simulink model "porte_avion_model"  (R2025a)
settings: Solver=VariableStepAuto  StartTime=0.0  StopTime=30  RelTol=1e-3
values from neighbouring files (symbols this model uses):
  a = 250e3    (= 250000)    [bateau_data.m]    (also in chariot_data.m; porte_avion.m)
  A = [0    1  0    0 ... (first row only)    [porte_avion.m]
  b = 1e9    (= 1000000000)    [bateau_data.m]    (also in chariot_data.m; porte_avion.m)
  B = [0 ... (first row only)    [porte_avion.m]
  c = 0.4e9    (= 400000000)    [bateau_data.m]    (also in chariot_data.m; porte_avion.m)
  C = [1 0 0 0 ... (first row only)    [porte_avion.m]
  d = 500e6    (= 500000000)    [bateau_data.m]    (also in chariot_data.m; porte_avion.m)
  D = [0 ... (first row only)    [porte_avion.m]
  f = 60    [bateau_data.m]    (also in chariot_data.m; porte_avion.m)
  g = 9.81    [bateau_data.m]    (also in chariot_data.m; porte_avion.m)
  theta_0 = pi/3    (= 1.0471975512)    [porte_avion.m]
  theta_dot_0 = 0    [porte_avion.m]
  x_0 = 0    [porte_avion.m]
  X_0 = [x_0 ... (first row only)    [porte_avion.m]
  x_dot_0 = 0    [porte_avion.m]
settings Model: Creator=vikfo  LastModifiedBy=vikfo

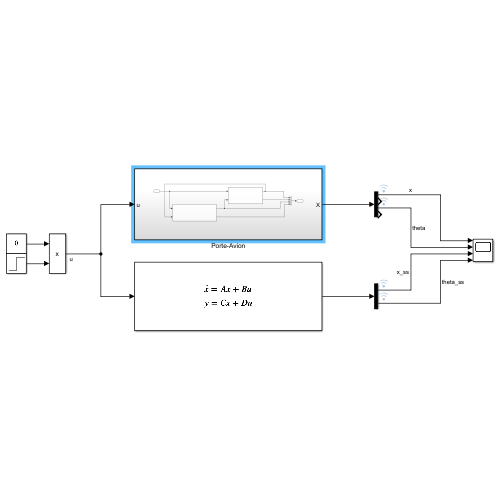
[thumbnail: Simulink's stored preview of the top-level diagram]
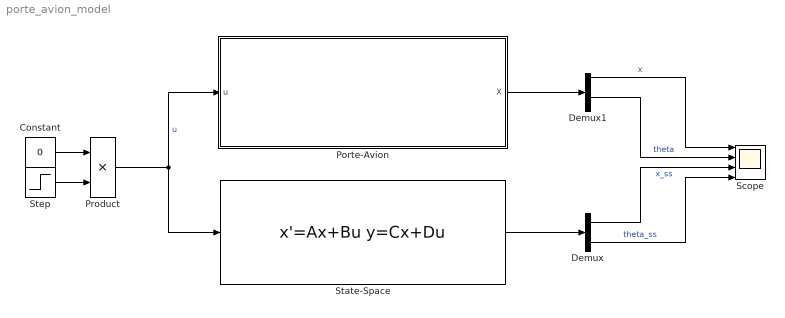
== system porte_avion_model ==
  Constant : Constant  Value=0
  Demux : Demux  Outputs=2
  Demux1 : Demux
  Porte-Avion : Subsystem
  Product : Product
  Scope : Scope  NumInputPorts=4
      settings: ActiveDisplayYMinimum=-1  ActiveDisplayYMaximum=1
  State-Space : StateSpace  A=A  B=B  C=C  D=D  InitialCondition=X_0
  Step : Step  SampleTime=0
  wires:
  Step/1 -> Product/2
  Constant/1 -> Product/1
  State-Space/1 -> Demux/1
  Demux/1 -> Scope/3  "x_ss"
  Product/1 -> Porte-Avion/1(u), State-Space/1  "u"
  Porte-Avion/1(X) -> Demux1/1
  Demux/2 -> Scope/4  "theta_ss"
  Demux1/1 -> Scope/1  "x"
  Demux1/3 -> Scope/2  "theta"

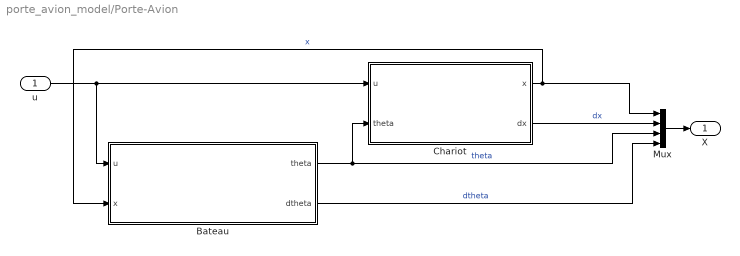
== system porte_avion_model/Porte-Avion ==
  u : Inport
  Bateau : Subsystem
  Chariot : Subsystem
  Mux : Mux
  X : Outport
  wires:
  Chariot/1(x) -> Bateau/2(x), Mux/1  "x"
  Bateau/1(theta) -> Mux/3, Chariot/2(theta)  "theta"
  Chariot/2(dx) -> Mux/2  "dx"
  u/1 -> Chariot/1(u), Bateau/1(u)
  Bateau/2(dtheta) -> Mux/4  "dtheta"
  Mux/1 -> X/1

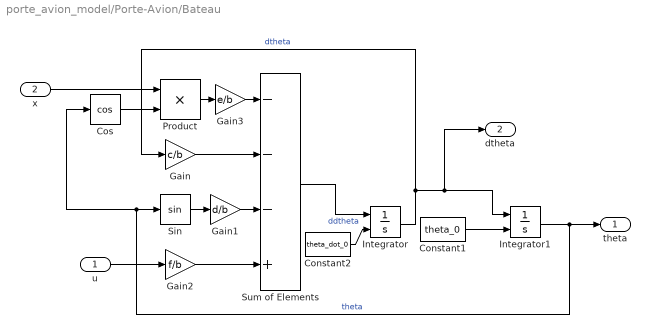
== system porte_avion_model/Porte-Avion/Bateau ==
  u : Inport
  x : Inport  Port=2
  Constant1 : Constant  Value=theta_0
  Constant2 : Constant  Value=theta_dot_0
  Cos : Trigonometry  Operator=cos
  Gain : Gain  Gain=c/b
  Gain1 : Gain  Gain=d/b
  Gain2 : Gain  Gain=f/b
  Gain3 : Gain  Gain=e/b
  Integrator : Integrator  InitialConditionSource=external
  Integrator1 : Integrator  InitialConditionSource=external
  Product : Product
  Sin : Trigonometry
  Sum of Elements : Sum  Inputs=---+
  theta : Outport
  dtheta : Outport  Port=2
  wires:
  Integrator/1 -> Gain/1, dtheta/1, Integrator1/1  "dtheta"
  u/1 -> Gain2/1
  Sum of Elements/1 -> Integrator/1  "ddtheta"
  Gain/1 -> Sum of Elements/2
  Gain2/1 -> Sum of Elements/4
  Integrator1/1 -> Cos/1, Sin/1, theta/1  "theta"
  Gain1/1 -> Sum of Elements/3
  Constant1/1 -> Integrator1/2
  Sin/1 -> Gain1/1
  Constant2/1 -> Integrator/2
  Gain3/1 -> Sum of Elements/1
  Product/1 -> Gain3/1
  x/1 -> Product/1
  Cos/1 -> Product/2

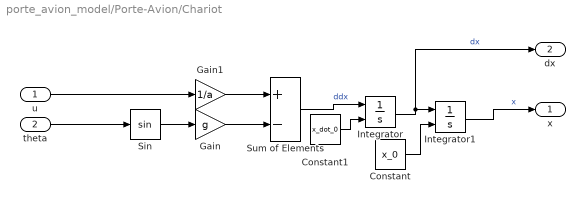
== system porte_avion_model/Porte-Avion/Chariot ==
  u : Inport
  theta : Inport  Port=2
  Constant : Constant  Value=x_0
  Constant1 : Constant  Value=x_dot_0
  Gain : Gain  Gain=g
  Gain1 : Gain  Gain=1/a
  Integrator : Integrator  InitialConditionSource=external
  Integrator1 : Integrator  InitialConditionSource=external
  Sin : Trigonometry
  Sum of Elements : Sum  Inputs=+-
  x : Outport
  dx : Outport  Port=2
  wires:
  Integrator/1 -> dx/1, Integrator1/1  "dx"
  Integrator1/1 -> x/1  "x"
  Sin/1 -> Gain/1
  Sum of Elements/1 -> Integrator/1  "ddx"
  Gain/1 -> Sum of Elements/2
  u/1 -> Gain1/1
  Gain1/1 -> Sum of Elements/1
  theta/1 -> Sin/1
  Constant/1 -> Integrator1/2
  Constant1/1 -> Integrator/2
